simulink model "lab7_MF"  (R2020a)
settings: Solver=FixedStepAuto  StartTime=0.0  StopTime=350  FixedStep=0.01  RelTol=1e-3
values from neighbouring files (symbols this model uses):
  a = max(abs(real([a1,a2])))    [pplane9.m]
  b = max(abs(imag([a1,a2])))    [pplane9.m]
  D = det(A)    [pplane9.m]
undefined symbols (not defined in the file or in its folder): A_2, g, h_bar, sigbuilder_block, u_bar
settings Model: Creator=bruno  LastModifiedBy=bruno

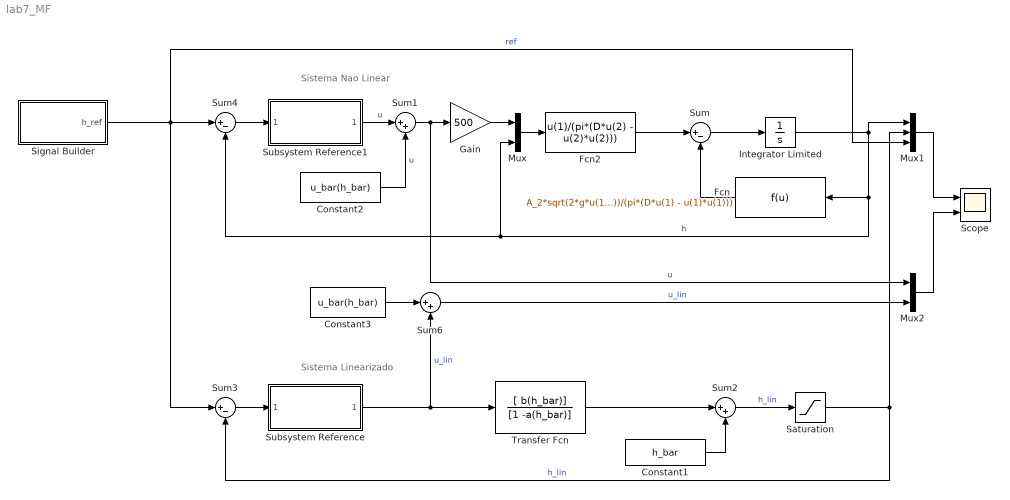
== system lab7_MF ==
  note: Sistema Linearizado
  note: Sistema Nao Linear
  Constant1 : Constant  Value=h_bar
  Constant2 : Constant  Value=u_bar(h_bar)
  Constant3 : Constant  Value=u_bar(h_bar)
  Fcn : Fcn  Expr=A_2*sqrt(2*g*u(1))/(pi*(D*u(1) - u(1)*u(1)))
  Fcn2 : Fcn  Expr=u(1)/(pi*(D*u(2) - u(2)*u(2)))
  Gain : Gain  Gain=500
  Integrator Limited : Integrator  InitialCondition=h_bar  LimitOutput=on  UpperSaturationLimit=100-0.001  LowerSaturationLimit=0.001
  Mux : Mux  Inputs=2
  Mux1 : Mux  Inputs=3
  Mux2 : Mux  Inputs=2
  Saturation : Saturate  UpperLimit=100 - 0.001  LowerLimit=0.001
  Scope : Scope  NumInputPorts=2
  Signal Builder : Subsystem  Tag=STV Subsys  LoadFcn=sigbuilder_block('load');  StartFcn=sigbuilder_block('start');  StopFcn=sigbuilder_block('stop');  ClipboardFcn=sigbuilder_block('clipboard');  mask(Sigbuilder block){tuvar=[0:10]}
      mask help: Simulink:masks:SigbuilderBlock_MD
      mask init:
      | if ~strcmp(get_param(bdroot(gcbh),'SimulationStatus'),'stopped') tuvar = sigbuilder_block('maskInit'); end
      settings: CopyFcn=sigbuilder_block('copy');  DeleteFcn=sigbuilder_block('delete');  ModelCloseFcn=sigbuilder_block('modelClose');  PreSaveFcn=sigbuilder_block('preSave');  PauseFcn=sigbuilder_block('pause');  ContinueFcn=sigbuilder_block('continue');  NameChangeFcn=sigbuilder_block('namechange');  OpenFcn=sigbuilder_block('open',[475.5 231.75 625.5 347.25 ]);  CloseFcn=sigbuilder_block('close');
      mask Display: plot(0, 0, 100, 100,[2, 2, 32, 32, 2], [68, 8, 8, 68, 68],[32, 2], [38, 38], [32, 19, 2],[53, 60, 44], [32, 17, 17, 2],[16, 16, 31, 31]);txt = getActiveGroup(gcbh);text(2, 100, txt,'verticalAlignment', 'top');
  Subsystem Reference : Subsystem  ReferencedSubsystem=PID_AW
  Subsystem Reference1 : Subsystem  ReferencedSubsystem=PID_AW
  Sum : Sum  Inputs=|+-
  Sum1 : Sum  Inputs=|++
  Sum2 : Sum  Inputs=|++
  Sum3 : Sum  Inputs=|+-
  Sum4 : Sum  Inputs=|+-
  Sum6 : Sum  Inputs=|++
  Transfer Fcn : TransferFcn  Numerator=[ b(h_bar)]  Denominator=[1 -a(h_bar)]
  wires:
  Sum/1 -> Integrator Limited/1
  Fcn2/1 -> Sum/1
  Fcn/1 -> Sum/2
  Sum1/1 -> Mux2/1, Gain/1  "u"
  Integrator Limited/1 -> Mux1/1, Fcn/1, Sum4/2, Mux/2  "h"
  Signal Builder/1(h_ref) -> Sum3/1, Mux1/3, Sum4/1  "ref"
  Gain/1 -> Mux/1
  Mux/1 -> Fcn2/1
  Constant1/1 -> Sum2/2
  Transfer Fcn/1 -> Sum2/1
  Mux1/1 -> Scope/1
  Saturation/1 -> Mux1/2, Sum3/2  "h_lin"
  Sum3/1 -> Subsystem Reference/1
  Subsystem Reference/1 -> Transfer Fcn/1, Sum6/2  "u_lin"
  Constant2/1 -> Sum1/2  "u"
  Subsystem Reference1/1 -> Sum1/1  "u"
  Sum4/1 -> Subsystem Reference1/1
  Mux2/1 -> Scope/2
  Constant3/1 -> Sum6/1
  Sum6/1 -> Mux2/2  "u_lin"
  Sum2/1 -> Saturation/1  "h_lin"

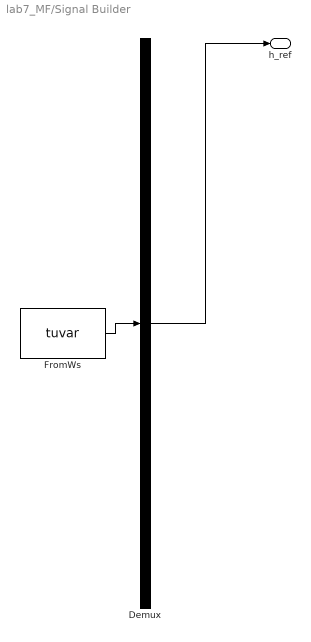
== system lab7_MF/Signal Builder ==
  Demux : Demux  Tag=STV Demux  Outputs=1
      settings: DisplayOption=none
  FromWs : FromWorkspace  Tag=STV FromWs  VariableName=tuvar
      SigBuilderData=|
      | common.afterFinalStr = 'Extrapolate'
      | common.sampleTime = 0
      | dataSet.timeRange = [0 350]
      | dataSet.name = 'Group 1'
      | sbobj.Groups.Name = 'Group 1'
      | sbobj.Groups.Signals.Name = 'h_ref'
      | sbobj.Groups.Signals.XData = [0 50 50 150 150 250 250 300 300 350]
      | sbobj.Groups.Signals.YData = [90 90 50 50 10 10 50 50 90 90]
      | sbobj.Groups.TimeRange = [0 350]
  h_ref : Outport  Tag=STV Outport
  wires:
  Demux/1 -> h_ref/1
  FromWs/1 -> Demux/1
